simulink model "taketwo_mode_sim"  (R2024a)
settings: Solver=FixedStepDiscrete  StartTime=0.0  StopTime=50.0  FixedStep=0.05  RelTol=1e-3
settings Model: Creator=katiegildersleeve  LastModifiedBy=katiegildersleeve

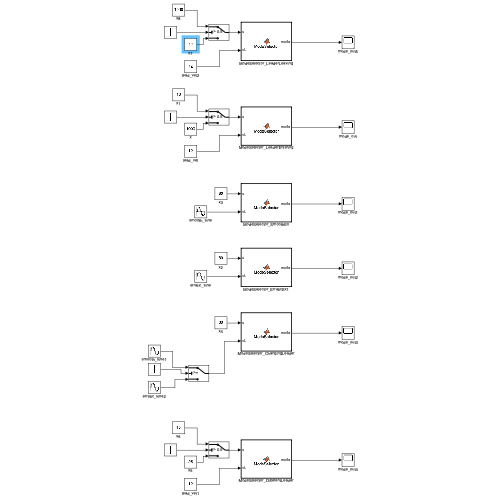
[thumbnail: Simulink's stored preview of the top-level diagram]
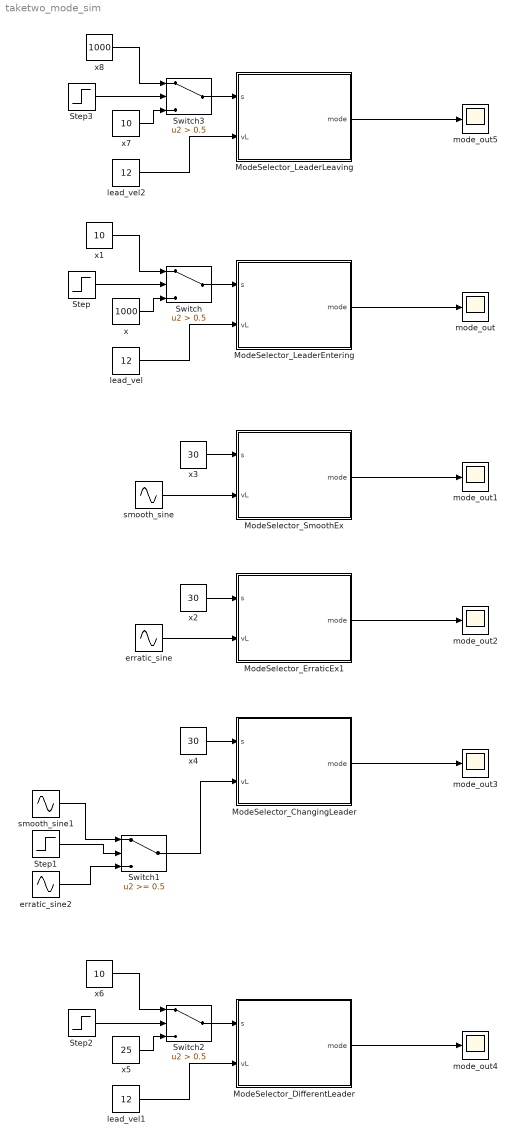
== system taketwo_mode_sim ==
  ModeSelector_ChangingLeader : MATLAB Function  TreatAsAtomicUnit=on
  ModeSelector_DifferentLeader : MATLAB Function  TreatAsAtomicUnit=on
  ModeSelector_ErraticEx1 : MATLAB Function  TreatAsAtomicUnit=on
  ModeSelector_LeaderEntering : MATLAB Function  TreatAsAtomicUnit=on
  ModeSelector_LeaderLeaving : MATLAB Function  TreatAsAtomicUnit=on
  ModeSelector_SmoothEx : MATLAB Function  TreatAsAtomicUnit=on
  Step : Step  Time=20  SampleTime=0
  Step1 : Step  Time=22
  Step2 : Step  Time=20  SampleTime=0
  Step3 : Step  Time=20  SampleTime=0
  Switch : Switch  Criteria=u2 > Threshold  Threshold=0.5  SaturateOnIntegerOverflow=off  InputSameDT=off
  Switch1 : Switch  Threshold=0.5  SaturateOnIntegerOverflow=off  InputSameDT=off
  Switch2 : Switch  Criteria=u2 > Threshold  Threshold=0.5  SaturateOnIntegerOverflow=off  InputSameDT=off
  Switch3 : Switch  Criteria=u2 > Threshold  Threshold=0.5  SaturateOnIntegerOverflow=off  InputSameDT=off
  erratic_sine : Sin  Amplitude=2.0  Bias=12  Frequency=0.5
  erratic_sine2 : Sin  Amplitude=2.0  Bias=12  Frequency=0.5
  lead_vel : Constant  Value=12
  lead_vel1 : Constant  Value=12
  lead_vel2 : Constant  Value=12
  mode_out{,1..5} (6 alike) : Scope
  smooth_sine : Sin  Amplitude=0.3  Bias=12  Frequency=0.2
  smooth_sine1 : Sin  Amplitude=0.3  Bias=12  Frequency=0.2
  x : Constant  Value=1000
  x1 : Constant  Value=10
  x2 : Constant  Value=30
  x3 : Constant  Value=30
  x4 : Constant  Value=30
  x5 : Constant  Value=25
  x6 : Constant  Value=10
  x7 : Constant  Value=10
  x8 : Constant  Value=1000
  wires:
  lead_vel/1 -> ModeSelector_LeaderEntering/2(vL)
  ModeSelector_LeaderEntering/1(mode) -> mode_out/1
  x/1 -> Switch/3
  Step/1 -> Switch/2
  Switch/1 -> ModeSelector_LeaderEntering/1(s)
  x1/1 -> Switch/1
  ModeSelector_SmoothEx/1(mode) -> mode_out1/1
  smooth_sine/1 -> ModeSelector_SmoothEx/2(vL)
  x3/1 -> ModeSelector_SmoothEx/1(s)
  erratic_sine/1 -> ModeSelector_ErraticEx1/2(vL)
  ModeSelector_ErraticEx1/1(mode) -> mode_out2/1
  x2/1 -> ModeSelector_ErraticEx1/1(s)
  Switch1/1 -> ModeSelector_ChangingLeader/2(vL)
  ModeSelector_ChangingLeader/1(mode) -> mode_out3/1
  x4/1 -> ModeSelector_ChangingLeader/1(s)
  erratic_sine2/1 -> Switch1/3
  smooth_sine1/1 -> Switch1/1
  Step1/1 -> Switch1/2
  ModeSelector_DifferentLeader/1(mode) -> mode_out4/1
  lead_vel1/1 -> ModeSelector_DifferentLeader/2(vL)
  x6/1 -> Switch2/1
  x5/1 -> Switch2/3
  Switch2/1 -> ModeSelector_DifferentLeader/1(s)
  Step2/1 -> Switch2/2
  ModeSelector_LeaderLeaving/1(mode) -> mode_out5/1
  lead_vel2/1 -> ModeSelector_LeaderLeaving/2(vL)
  x8/1 -> Switch3/1
  x7/1 -> Switch3/3
  Switch3/1 -> ModeSelector_LeaderLeaving/1(s)
  Step3/1 -> Switch3/2

== matlab function taketwo_mode_sim/ModeSelector_LeaderEntering ==
  data: s input; mode output; vL input
function mode = ModeSelector(s, vL)
% 1 = no leader (s>50)
% 2 = collecting (warm-up)
% 3 = smooth leader (after warm-up)
% 4 = erratic leader (after warm-up)

%#codegen
% ---------- Tunables ----------
Ts               = 0.05;   % match model fixed-step
S_NOLEADER       = 50.0;   % [m]
COLLECT_SECS     = 15.0;   % [s]
S_JUMP_THR       = 15.0;   % [m]
EWMA_TAU         = 3.0;    % [s]
SIGMA_LOW        = 0.50;   % [m/s]
SIGMA_HIGH       = 0.80;   % [m/s]
% --------------------------------

persistent inited prev_s prev_present collect_cnt mu var last_mode
if isempty(inited)
    inited        = true;
    prev_s        = s;
    prev_present  = (s <= S_NOLEADER);
    % *** Force warm-up if a leader is present at t=0 ***
    collect_cnt   = int32( prev_present * round(COLLECT_SECS / Ts) );
    mu            = vL;
    var           = 0.0;
    last_mode     = uint8(1);
end

leader_present = (s <= S_NOLEADER);

% (A) start warm-up when leader first appears (no->yes)
if leader_present && ~prev_present
    collect_cnt = int32(round(COLLECT_SECS / Ts));
    mu = vL; var = 0.0;
end

% (B) restart warm-up on any large one-sample space-gap jump
ds = s - prev_s;
if abs(ds) >= S_JUMP_THR
    collect_cnt = int32(round(COLLECT_SECS / Ts));
    mu = vL; var = 0.0;
end

% EWMA update only when leader present
alpha = Ts / max(EWMA_TAU, Ts); if alpha > 1, alpha = 1; end
if leader_present
    mu  = (1 - alpha)*mu + alpha*vL;
    d   = vL - mu;
    var = (1 - alpha)*(var + alpha*d*d);
else
    mu = vL; var = 0.0;
end
sigma = sqrt(max(var,0.0));

% ----- Mode decision -----
if ~leader_present
    mode = uint8(1);
else
    if collect_cnt > 0
        collect_cnt = collect_cnt - 1;
        mode = uint8(2);              % *** hold Mode 2 during warm-up ***
    else
        % hysteresis classification after warm-up
        if last_mode == uint8(4)
            mode = uint8( sigma <= SIGMA_LOW ) * 3 + uint8( sigma > SIGMA_LOW ) * 4;
        else
            mode = uint8( sigma >= SIGMA_HIGH ) * 4 + uint8( sigma < SIGMA_HIGH ) * 3;
        end
    end
end

% Bookkeeping
last_mode    = mode;
prev_s       = s;
prev_present = leader_present;

== matlab function taketwo_mode_sim/ModeSelector_ErraticEx1 ==
  data: s input; mode output; vL input
function mode = ModeSelector(s, vL)
% 1 = no leader (s>50)
% 2 = collecting (warm-up)
% 3 = smooth leader (after warm-up)
% 4 = erratic leader (after warm-up)

%#codegen
% ---------- Tunables ----------
Ts               = 0.05;   % match model fixed-step
S_NOLEADER       = 50.0;   % [m]
COLLECT_SECS     = 15.0;   % [s]
S_JUMP_THR       = 15.0;   % [m]
EWMA_TAU         = 3.0;    % [s]
SIGMA_LOW        = 0.50;   % [m/s]
SIGMA_HIGH       = 0.80;   % [m/s]
% --------------------------------

persistent inited prev_s prev_present collect_cnt mu var last_mode
if isempty(inited)
    inited        = true;
    prev_s        = s;
    prev_present  = (s <= S_NOLEADER);
    % *** Force warm-up if a leader is present at t=0 ***
    collect_cnt   = int32( prev_present * round(COLLECT_SECS / Ts) );
    mu            = vL;
    var           = 0.0;
    last_mode     = uint8(1);
end

leader_present = (s <= S_NOLEADER);

% (A) start warm-up when leader first appears (no->yes)
if leader_present && ~prev_present
    collect_cnt = int32(round(COLLECT_SECS / Ts));
    mu = vL; var = 0.0;
end

% (B) restart warm-up on any large one-sample space-gap jump
ds = s - prev_s;
if abs(ds) >= S_JUMP_THR
    collect_cnt = int32(round(COLLECT_SECS / Ts));
    mu = vL; var = 0.0;
end

% EWMA update only when leader present
alpha = Ts / max(EWMA_TAU, Ts); if alpha > 1, alpha = 1; end
if leader_present
    mu  = (1 - alpha)*mu + alpha*vL;
    d   = vL - mu;
    var = (1 - alpha)*(var + alpha*d*d);
else
    mu = vL; var = 0.0;
end
sigma = sqrt(max(var,0.0));

% ----- Mode decision -----
if ~leader_present
    mode = uint8(1);
else
    if collect_cnt > 0
        collect_cnt = collect_cnt - 1;
        mode = uint8(2);              % *** hold Mode 2 during warm-up ***
    else
        % hysteresis classification after warm-up
        if last_mode == uint8(4)
            mode = uint8( sigma <= SIGMA_LOW ) * 3 + uint8( sigma > SIGMA_LOW ) * 4;
        else
            mode = uint8( sigma >= SIGMA_HIGH ) * 4 + uint8( sigma < SIGMA_HIGH ) * 3;
        end
    end
end

% Bookkeeping
last_mode    = mode;
prev_s       = s;
prev_present = leader_present;

== matlab function taketwo_mode_sim/ModeSelector_ChangingLeader ==
  data: s input; mode output; vL input
function mode = ModeSelector(s, vL)
% 1 = no leader (s>50)
% 2 = collecting (warm-up)
% 3 = smooth leader (after warm-up)
% 4 = erratic leader (after warm-up)

%#codegen
% ---------- Tunables ----------
Ts               = 0.05;   % match model fixed-step
S_NOLEADER       = 50.0;   % [m]
COLLECT_SECS     = 15.0;   % [s]
S_JUMP_THR       = 15.0;   % [m]
EWMA_TAU         = 3.0;    % [s]
SIGMA_LOW        = 0.50;   % [m/s]
SIGMA_HIGH       = 0.80;   % [m/s]
% --------------------------------

persistent inited prev_s prev_present collect_cnt mu var last_mode
if isempty(inited)
    inited        = true;
    prev_s        = s;
    prev_present  = (s <= S_NOLEADER);
    % *** Force warm-up if a leader is present at t=0 ***
    collect_cnt   = int32( prev_present * round(COLLECT_SECS / Ts) );
    mu            = vL;
    var           = 0.0;
    last_mode     = uint8(1);
end

leader_present = (s <= S_NOLEADER);

% (A) start warm-up when leader first appears (no->yes)
if leader_present && ~prev_present
    collect_cnt = int32(round(COLLECT_SECS / Ts));
    mu = vL; var = 0.0;
end

% (B) restart warm-up on any large one-sample space-gap jump
ds = s - prev_s;
if abs(ds) >= S_JUMP_THR
    collect_cnt = int32(round(COLLECT_SECS / Ts));
    mu = vL; var = 0.0;
end

% EWMA update only when leader present
alpha = Ts / max(EWMA_TAU, Ts); if alpha > 1, alpha = 1; end
if leader_present
    mu  = (1 - alpha)*mu + alpha*vL;
    d   = vL - mu;
    var = (1 - alpha)*(var + alpha*d*d);
else
    mu = vL; var = 0.0;
end
sigma = sqrt(max(var,0.0));

% ----- Mode decision -----
if ~leader_present
    mode = uint8(1);
else
    if collect_cnt > 0
        collect_cnt = collect_cnt - 1;
        mode = uint8(2);              % *** hold Mode 2 during warm-up ***
    else
        % hysteresis classification after warm-up
        if last_mode == uint8(4)
            mode = uint8( sigma <= SIGMA_LOW ) * 3 + uint8( sigma > SIGMA_LOW ) * 4;
        else
            mode = uint8( sigma >= SIGMA_HIGH ) * 4 + uint8( sigma < SIGMA_HIGH ) * 3;
        end
    end
end

% Bookkeeping
last_mode    = mode;
prev_s       = s;
prev_present = leader_present;

== matlab function taketwo_mode_sim/ModeSelector_DifferentLeader ==
  data: s input; mode output; vL input
function mode = ModeSelector(s, vL)
% 1 = no leader (s>50)
% 2 = collecting (warm-up)
% 3 = smooth leader (after warm-up)
% 4 = erratic leader (after warm-up)

%#codegen
% ---------- Tunables ----------
Ts               = 0.05;   % match model fixed-step
S_NOLEADER       = 50.0;   % [m]
COLLECT_SECS     = 15.0;   % [s]
S_JUMP_THR       = 15.0;   % [m]
EWMA_TAU         = 3.0;    % [s]
SIGMA_LOW        = 0.50;   % [m/s]
SIGMA_HIGH       = 0.80;   % [m/s]
% --------------------------------

persistent inited prev_s prev_present collect_cnt mu var last_mode
if isempty(inited)
    inited        = true;
    prev_s        = s;
    prev_present  = (s <= S_NOLEADER);
    % *** Force warm-up if a leader is present at t=0 ***
    collect_cnt   = int32( prev_present * round(COLLECT_SECS / Ts) );
    mu            = vL;
    var           = 0.0;
    last_mode     = uint8(1);
end

leader_present = (s <= S_NOLEADER);

% (A) start warm-up when leader first appears (no->yes)
if leader_present && ~prev_present
    collect_cnt = int32(round(COLLECT_SECS / Ts));
    mu = vL; var = 0.0;
end

% (B) restart warm-up on any large one-sample space-gap jump
ds = s - prev_s;
if abs(ds) >= S_JUMP_THR
    collect_cnt = int32(round(COLLECT_SECS / Ts));
    mu = vL; var = 0.0;
end

% EWMA update only when leader present
alpha = Ts / max(EWMA_TAU, Ts); if alpha > 1, alpha = 1; end
if leader_present
    mu  = (1 - alpha)*mu + alpha*vL;
    d   = vL - mu;
    var = (1 - alpha)*(var + alpha*d*d);
else
    mu = vL; var = 0.0;
end
sigma = sqrt(max(var,0.0));

% ----- Mode decision -----
if ~leader_present
    mode = uint8(1);
else
    if collect_cnt > 0
        collect_cnt = collect_cnt - 1;
        mode = uint8(2);              % *** hold Mode 2 during warm-up ***
    else
        % hysteresis classification after warm-up
        if last_mode == uint8(4)
            mode = uint8( sigma <= SIGMA_LOW ) * 3 + uint8( sigma > SIGMA_LOW ) * 4;
        else
            mode = uint8( sigma >= SIGMA_HIGH ) * 4 + uint8( sigma < SIGMA_HIGH ) * 3;
        end
    end
end

% Bookkeeping
last_mode    = mode;
prev_s       = s;
prev_present = leader_present;

== matlab function taketwo_mode_sim/ModeSelector_LeaderLeaving ==
  data: s input; mode output; vL input
function mode = ModeSelector(s, vL)
% 1 = no leader (s>50)
% 2 = collecting (warm-up)
% 3 = smooth leader (after warm-up)
% 4 = erratic leader (after warm-up)

%#codegen
% ---------- Tunables ----------
Ts               = 0.05;   % match model fixed-step
S_NOLEADER       = 50.0;   % [m]
COLLECT_SECS     = 15.0;   % [s]
S_JUMP_THR       = 15.0;   % [m]
EWMA_TAU         = 3.0;    % [s]
SIGMA_LOW        = 0.50;   % [m/s]
SIGMA_HIGH       = 0.80;   % [m/s]
% --------------------------------

persistent inited prev_s prev_present collect_cnt mu var last_mode
if isempty(inited)
    inited        = true;
    prev_s        = s;
    prev_present  = (s <= S_NOLEADER);
    % *** Force warm-up if a leader is present at t=0 ***
    collect_cnt   = int32( prev_present * round(COLLECT_SECS / Ts) );
    mu            = vL;
    var           = 0.0;
    last_mode     = uint8(1);
end

leader_present = (s <= S_NOLEADER);

% (A) start warm-up when leader first appears (no->yes)
if leader_present && ~prev_present
    collect_cnt = int32(round(COLLECT_SECS / Ts));
    mu = vL; var = 0.0;
end

% (B) restart warm-up on any large one-sample space-gap jump
ds = s - prev_s;
if abs(ds) >= S_JUMP_THR
    collect_cnt = int32(round(COLLECT_SECS / Ts));
    mu = vL; var = 0.0;
end

% EWMA update only when leader present
alpha = Ts / max(EWMA_TAU, Ts); if alpha > 1, alpha = 1; end
if leader_present
    mu  = (1 - alpha)*mu + alpha*vL;
    d   = vL - mu;
    var = (1 - alpha)*(var + alpha*d*d);
else
    mu = vL; var = 0.0;
end
sigma = sqrt(max(var,0.0));

% ----- Mode decision -----
if ~leader_present
    mode = uint8(1);
else
    if collect_cnt > 0
        collect_cnt = collect_cnt - 1;
        mode = uint8(2);              % *** hold Mode 2 during warm-up ***
    else
        % hysteresis classification after warm-up
        if last_mode == uint8(4)
            mode = uint8( sigma <= SIGMA_LOW ) * 3 + uint8( sigma > SIGMA_LOW ) * 4;
        else
            mode = uint8( sigma >= SIGMA_HIGH ) * 4 + uint8( sigma < SIGMA_HIGH ) * 3;
        end
    end
end

% Bookkeeping
last_mode    = mode;
prev_s       = s;
prev_present = leader_present;

== matlab function taketwo_mode_sim/ModeSelector_SmoothEx ==
  data: s input; mode output; vL input
function mode = ModeSelector(s, vL)
% 1 = no leader (s>50)
% 2 = collecting (warm-up)
% 3 = smooth leader (after warm-up)
% 4 = erratic leader (after warm-up)

%#codegen
% ---------- Tunables ----------
Ts               = 0.05;   % match model fixed-step
S_NOLEADER       = 50.0;   % [m]
COLLECT_SECS     = 15.0;   % [s]
S_JUMP_THR       = 15.0;   % [m]
EWMA_TAU         = 3.0;    % [s]
SIGMA_LOW        = 0.50;   % [m/s]
SIGMA_HIGH       = 0.80;   % [m/s]
% --------------------------------

persistent inited prev_s prev_present collect_cnt mu var last_mode
if isempty(inited)
    inited        = true;
    prev_s        = s;
    prev_present  = (s <= S_NOLEADER);
    % *** Force warm-up if a leader is present at t=0 ***
    collect_cnt   = int32( prev_present * round(COLLECT_SECS / Ts) );
    mu            = vL;
    var           = 0.0;
    last_mode     = uint8(1);
end

leader_present = (s <= S_NOLEADER);

% (A) start warm-up when leader first appears (no->yes)
if leader_present && ~prev_present
    collect_cnt = int32(round(COLLECT_SECS / Ts));
    mu = vL; var = 0.0;
end

% (B) restart warm-up on any large one-sample space-gap jump
ds = s - prev_s;
if abs(ds) >= S_JUMP_THR
    collect_cnt = int32(round(COLLECT_SECS / Ts));
    mu = vL; var = 0.0;
end

% EWMA update only when leader present
alpha = Ts / max(EWMA_TAU, Ts); if alpha > 1, alpha = 1; end
if leader_present
    mu  = (1 - alpha)*mu + alpha*vL;
    d   = vL - mu;
    var = (1 - alpha)*(var + alpha*d*d);
else
    mu = vL; var = 0.0;
end
sigma = sqrt(max(var,0.0));

% ----- Mode decision -----
if ~leader_present
    mode = uint8(1);
else
    if collect_cnt > 0
        collect_cnt = collect_cnt - 1;
        mode = uint8(2);              % *** hold Mode 2 during warm-up ***
    else
        % hysteresis classification after warm-up
        if last_mode == uint8(4)
            mode = uint8( sigma <= SIGMA_LOW ) * 3 + uint8( sigma > SIGMA_LOW ) * 4;
        else
            mode = uint8( sigma >= SIGMA_HIGH ) * 4 + uint8( sigma < SIGMA_HIGH ) * 3;
        end
    end
end

% Bookkeeping
last_mode    = mode;
prev_s       = s;
prev_present = leader_present;
